simulink model "rebi"  (Simulink 7.6)
settings: Solver=ode1  StartTime=0.0  StopTime=10  FixedStep=0.001  RelTol=1e-3
PostLoadFcn:
  | , if any(exist('dsrtsu_mdlpostloadfcn', 'file') == [2, 3, 6]), try dsrtsu_mdlpostloadfcn('Execute', bdroot); catch fprintf('Error in PostLoadFcn (dsrtsu_mdlpostloadfcn) for model "%s":\n %s\n', bdroot, lasterr); end, end,
values from neighbouring files (symbols this model uses):
  A = [0 1 ; -w0^2 -2*xhi*w0]    [integral_state_feedback_pole_placement.m]    (also in lqr_integral_control.m = [-2*xhi*omega0  -omega0^2  0     0           0)
  B = [0 ; k*w0]    [integral_state_feedback_pole_placement.m]    (also in lqr_integral_control.m = [Ke*omega0^2     Ke*omega0^2)
  C = [1 0]    [integral_state_feedback_pole_placement.m]    (also in lqr_integral_control.m = [0 1 0 0 0)
  Ki = K(:, n+1:n+p)    [lqr_integral_control.m]
  Kp = K(:, 1:n)    [lqr_integral_control.m]
settings Model: DSRTSU_INTERNAL_RTI_VER=370  DSRTSU_INTERNAL_RTI_TYPE=rti1104  Creator=eleve  LastModifiedBy=eleve  BufferReuse=off
settings OptimizationCC: BlockReduction=off  OptimizeBlockIOStorage=off  BufferReuse=off  ExpressionFolding=off  LocalBlockOutputs=off
settings HardwareCC: ProdIntDivRoundTo=Zero  ProdEndianess=BigEndian  ProdHWDeviceType=Generic->Custom  TargetIntDivRoundTo=Zero  TargetEndianess=BigEndian  TargetHWDeviceType=Generic->Custom
settings RTWCC: SystemTargetFile=rti1104.tlc  MakeCommand=make_rti  TemplateMakefile=rti1104.tmf  Description=dSPACE DS1104 Hardware Platform  ProcessScript=rti1104_make_rtw_hook
settings STFCustomTargetCC: ParMdlRefBuildCompliant=on  GeneratePreprocessorConditionals=Disable all  SystemTargetFile=rti1104.tlc
settings GRTTargetCC: CompOptLevelCompliant=off  MatFileLogging=off  ExtModeMexFile=noextcomm
settings CustomProperty: DataType=RTWOptions_EnumType_C__dSPACE_matlab_rti1104_tlc_rti1104_1InitialSimState  Value=RUN
settings EnumStrPairs: String=RUN

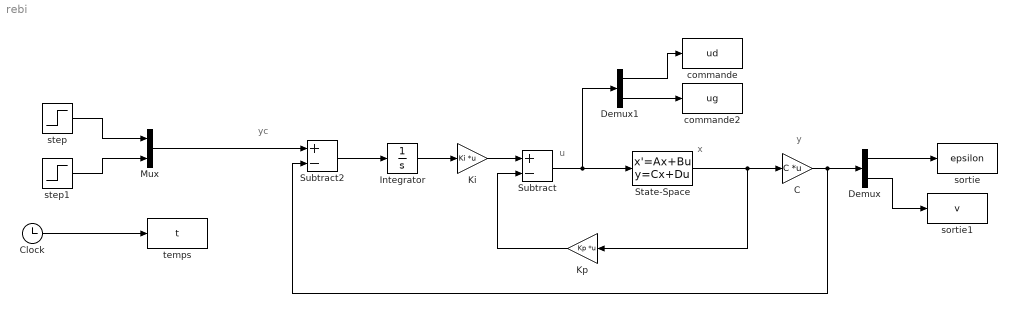
== system rebi ==
  note: u
  note: yc
  note: x
  note: y
  C : Gain  Gain=C  Multiplication=Matrix(K*u) (u vector)
  Clock : Clock
      settings: Decimation=10
  Demux : Demux  Outputs=2
  Demux1 : Demux  Outputs=2
  Integrator : Integrator
  Ki : Gain  Gain=Ki  Multiplication=Matrix(K*u) (u vector)
  Kp : Gain  Gain=Kp  Multiplication=Matrix(K*u) (u vector)
  Mux : Mux  Inputs=2
  State-Space : StateSpace  A=A  B=B  C=eye(5)  D=zeros(5,2)
  Subtract : Sum  Inputs=+-
  Subtract2 : Sum  Inputs=+-
  commande : ToWorkspace  VariableName=ud  SampleTime=-1  SaveFormat=Array
  commande2 : ToWorkspace  VariableName=ug  SampleTime=-1  SaveFormat=Array
  sortie : ToWorkspace  VariableName=epsilon  SampleTime=-1  SaveFormat=Array
  sortie1 : ToWorkspace  VariableName=v  SampleTime=-1  SaveFormat=Array
  step : Step  After=pi/6  SampleTime=0
  step1 : Step  SampleTime=0
  temps : ToWorkspace  VariableName=t  SampleTime=-1  SaveFormat=Array
  wires:
  Subtract2/1 -> Integrator/1
  Integrator/1 -> Ki/1
  Ki/1 -> Subtract/1
  Kp/1 -> Subtract/2
  Subtract/1 -> State-Space/1, Demux1/1
  State-Space/1 -> Kp/1, C/1
  Clock/1 -> temps/1
  C/1 -> Subtract2/2, Demux/1
  Demux/1 -> sortie/1
  Demux/2 -> sortie1/1
  Demux1/1 -> commande/1
  Demux1/2 -> commande2/1
  step/1 -> Mux/1
  step1/1 -> Mux/2
  Mux/1 -> Subtract2/1
